simulink model "DSBb"  (R2013b)
settings: Solver=ode45  StartTime=0.0  StopTime=10.0  RelTol=1e-3
libraries: dspsrcs4 x1
settings Model: Creator=Nouri  LastModifiedBy=Nouri

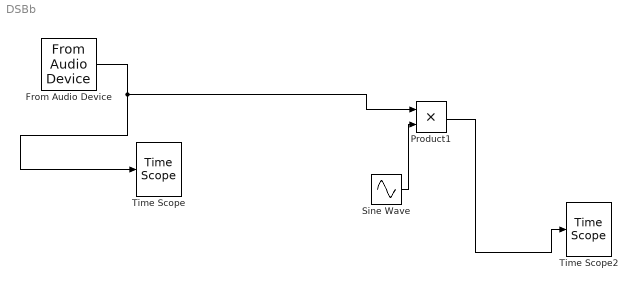
== system DSBb ==
  From Audio Device : dspsrcs4/From Audio Device  deviceName=Default  numChannels=1  sampleRate=44000  deviceDatatype=Determine from output data type  autoBufferSize=on  bufferSize=4096  queueDuration=5  frameSize=1  outputDatatype=single  defaultInputChannelMapping=on  inputChannelMapping=1:2
  Product1 : Product
  Sine Wave : Sin  Amplitude=5  Frequency=88000  SampleTime=0
  Time Scope : TimeScope  DefaultConfigurationName=spbscopes.TimeScopeBlockCfg
      settings: CopyFcn=scopeextensions.ScopeBlock.onCoreBlockCopy(gcbh);  DeleteFcn=scopeextensions.ScopeBlock.callback(gcbh, 'onBlockDelete');  PreSaveFcn=scopeextensions.ScopeBlock.callback(gcbh, 'onModelSave');  NameChangeFcn=scopeextensions.ScopeBlock.callback(gcbh, 'onBlockRename');  DestroyFcn=scopeextensions.ScopeBlock.onBlockDestroy(gcbh)  CloseFcn=scopeextensions.ScopeBlock.callback(gcbh, 'onBlockClose');  PreDeleteFcn=scopeextensions.ScopeBlock.callback(gcbh, 'onBlockPreDelete');
  Time Scope2 : TimeScope  DefaultConfigurationName=spbscopes.TimeScopeBlockCfg
      settings: CopyFcn=scopeextensions.ScopeBlock.onCoreBlockCopy(gcbh);  DeleteFcn=scopeextensions.ScopeBlock.callback(gcbh, 'onBlockDelete');  PreSaveFcn=scopeextensions.ScopeBlock.callback(gcbh, 'onModelSave');  NameChangeFcn=scopeextensions.ScopeBlock.callback(gcbh, 'onBlockRename');  DestroyFcn=scopeextensions.ScopeBlock.onBlockDestroy(gcbh)  CloseFcn=scopeextensions.ScopeBlock.callback(gcbh, 'onBlockClose');  PreDeleteFcn=scopeextensions.ScopeBlock.callback(gcbh, 'onBlockPreDelete');
  wires:
  Sine Wave/1 -> Product1/2
  Product1/1 -> Time Scope2/1
  From Audio Device/1 -> Product1/1, Time Scope/1
